simulink model "gm_sampleModel1432_2_sub_sub"  (R2023a)
settings: Solver=VariableStepAuto  StartTime=0.0  StopTime=10.0  RelTol=1e-3
libraries: simulink x1, hdlsllib x1
settings Model: Creator=user1  LastModifiedBy=user1
settings OptimizationCC: BlockReduction=off  ConditionallyExecuteInputs=off
settings DebuggingCC: InheritedTsInSrcMsg=none

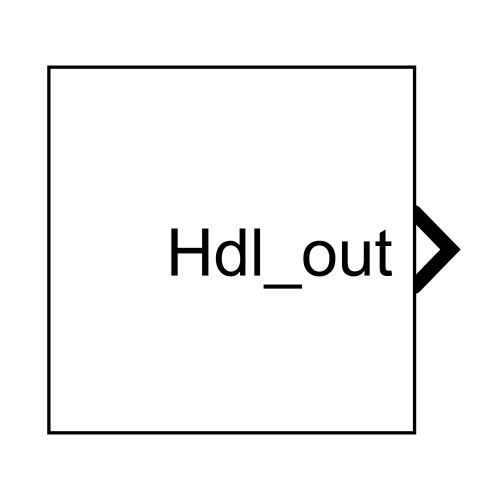
[thumbnail: Simulink's stored preview of the top-level diagram]
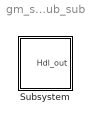
== system gm_sampleModel1432_2_sub_sub ==
  Subsystem : Subsystem

== system gm_sampleModel1432_2_sub_sub/Subsystem ==
  Subsystem : Subsystem
  Hdl_out : Outport  OutDataTypeStr=uint8  SampleTime=1
  wires:
  Subsystem/1(Hdl_out) -> Hdl_out/1

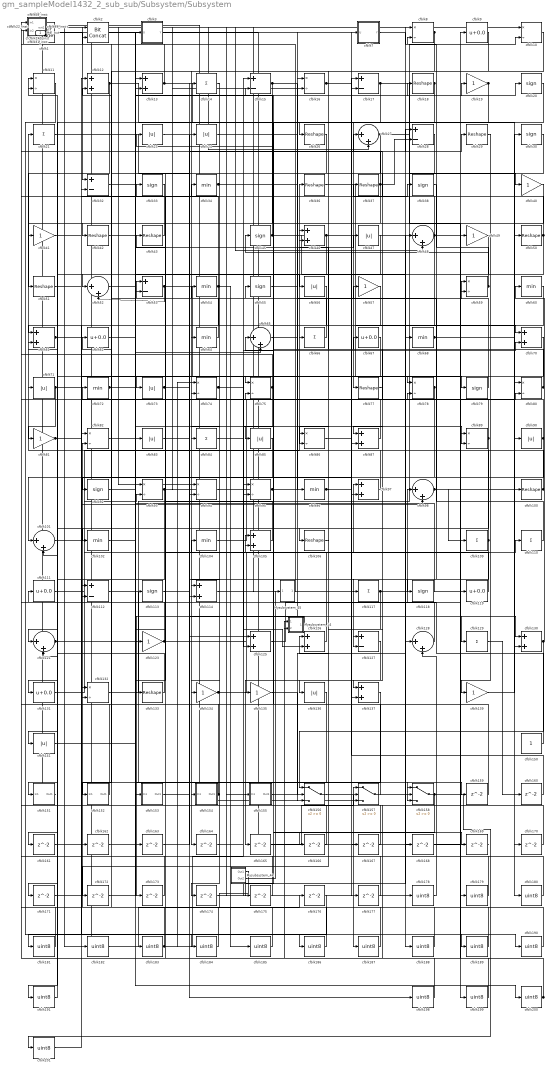
== system gm_sampleModel1432_2_sub_sub/Subsystem/Subsystem ==
  Mysubsystem_14 : Subsystem
  Mysubsystem_44 : Subsystem
  Mysubsystem_45 : Subsystem
  cfblk1 : simulink/Logic and Bit Operations/Detect Change  vinit=0  OutDataTypeStr=uint8
      settings: LibrarySourceBlock=|
      | hdlsllib/Logic and Bit
      | Operations/Detect
      | Change
  cfblk{8,10..11,16,59,74..75,78,80,82,86,89,93..95,132} (16 alike) : Product  Inputs=*/  OutDataTypeStr=uint8  RndMeth=Zero  SaturateOnIntegerOverflow=on
  cfblk{18,26,29,36..37,42..43,50..51,77,100,106,133} (13 alike) : Reshape
  cfblk{27,48,52,65,98,101,121,128} (8 alike) : Sum  Inputs=|++  OutDataTypeStr=uint8
  cfblk{34,54,60,64,68,72,96,102,104} (9 alike) : MinMax  OutDataTypeStr=uint8
  cfblk{12..13,46,61,70,87,97,105,114,125..126,130,137} (13 alike) : Sum  OutDataTypeStr=uint8
  cfblk107_inst : Subsystem
  cfblk108_inst : Subsystem
  cfblk{14,21,66,84,109..110,117,129} (8 alike) : Sum  Inputs=+  OutDataTypeStr=uint8
  cfblk{9,62,67,111,119,131} (6 alike) : Bias  Bias=0.0  SaturateOnIntegerOverflow=off
  cfblk{15,17,28,32,53,112,127} (7 alike) : Sum  Inputs=+-  OutDataTypeStr=uint8
  cfblk{20,30,33,38,45,55,79,92,113,118} (10 alike) : Signum
  cfblk120_inst : Subsystem
  cfblk122_inst : Subsystem
  cfblk{19,40..41,49,57,81,123,134..135,139} (10 alike) : Gain  OutDataTypeStr=uint8
  cfblk{23..24,47,56,71,73,83,85,90,136,141} (11 alike) : Abs  OutDataTypeStr=uint8  SaturateOnIntegerOverflow=off
  cfblk138_inst : Subsystem
  cfblk140_inst : Subsystem
  cfblk150 : Constant  OutDataTypeStr=uint8  SampleTime=-1
  cfblk151 : Subsystem
  cfblk152 : Subsystem
  cfblk153 : Subsystem
  cfblk154 : Subsystem
  cfblk155 : Subsystem
  cfblk156 : Switch  OutDataTypeStr=uint8  SaturateOnIntegerOverflow=off  InputSameDT=off
  cfblk157 : Switch  OutDataTypeStr=uint8  SaturateOnIntegerOverflow=off  InputSameDT=off
  cfblk158 : Switch  OutDataTypeStr=uint8  SaturateOnIntegerOverflow=off  InputSameDT=off
  cfblk{159..177} (19 alike) : Delay  SampleTime=1
  cfblk{178..191,198..201} (18 alike) : DataTypeConversion  OutDataTypeStr=uint8  SaturateOnIntegerOverflow=off  RndMeth=Floor
  cfblk2 : hdlsllib/Logic and Bit Operations/Bit Concat  numInputs=2
  cfblk22_inst : Subsystem
  cfblk3 : Subsystem  mask(Detect Rise Positive){vinit=double(0), InputProcessing=Elements as channels (sample based), OutDataTypeStr=uint8}
      mask prompts: vinit "Simulink:masks:InitialCondition_MP"; InputProcessing "Simulink:masks:InputProcessing_MP"; OutDataTypeStr "Simulink:masks:OutputDataType_MP"
      mask help: Simulink:masks:DetectRisePositive_MD
      mask init:
      | InputProcessing = 'Elements as channels (sample based)';
      | OutDataTypeStr = 'uint8';
      | vinit = double(0);
      mask TypeOptions InputProcessing: Simulink:masks:ColumnsAsChannelsFrameBased | Simulink:masks:ElementsAsChannelsSampleBased
      mask TypeOptions OutDataTypeStr: Simulink:masks:uint8 | Simulink:masks:boolean
      mask Display: fprintf('U > 0\n&  NOT\nU/z > 0')
  cfblk31_inst : Subsystem
  cfblk5 : Constant  Value=0  OutDataTypeStr=uint8  SampleTime=1
  cfblk58_inst : Subsystem
  cfblk7 : Subsystem  mask(Detect Fall Negative){vinit=double(0), InputProcessing=Elements as channels (sample based), OutDataTypeStr=uint8}
      mask prompts: vinit "Simulink:masks:InitialCondition_MP"; InputProcessing "Simulink:masks:InputProcessing_MP"; OutDataTypeStr "Simulink:masks:OutputDataType_MP"
      mask help: Simulink:masks:DetectFallNegative_MD
      mask init:
      | InputProcessing = 'Elements as channels (sample based)';
      | OutDataTypeStr = 'uint8';
      | vinit = double(0);
      mask TypeOptions InputProcessing: Simulink:masks:ColumnsAsChannelsFrameBased | Simulink:masks:ElementsAsChannelsSampleBased
      mask TypeOptions OutDataTypeStr: Simulink:masks:uint8 | Simulink:masks:boolean
      mask Display: fprintf('U < 0\n&  NOT\nU/z < 0')
  cfblk99_inst : Subsystem
  Hdl_out : Outport  OutDataTypeStr=uint8  SampleTime=1
  wires:
  Mysubsystem_14/1(Out1) -> cfblk173/1
  Mysubsystem_44/1(Out1) -> cfblk82/2
  Mysubsystem_44/2(Out2) -> Mysubsystem_45/1(In1)
  Mysubsystem_45/1(Out1) -> cfblk140_inst/2(in2)
  cfblk1/1 -> cfblk32/1
  cfblk10/1 -> cfblk164/1
  cfblk100/1 -> cfblk36/1, cfblk21/1
  cfblk101/1 -> cfblk93/2
  cfblk102/1 -> cfblk3/1(U)
  cfblk104/1 -> cfblk80/2
  cfblk105/1 -> cfblk53/1
  cfblk106/1 -> cfblk126/1
  cfblk107_inst/1(out1) -> cfblk27/2, cfblk119/1
  cfblk108_inst/1(out1) -> cfblk94/1
  cfblk109/1 -> cfblk62/1, cfblk127/2
  cfblk11/1 -> cfblk189/1
  cfblk110/1 -> cfblk55/1
  cfblk111/1 -> cfblk105/1
  cfblk112/1 -> cfblk154/1(In1)
  cfblk113/1 -> cfblk24/1
  cfblk114/1 -> cfblk169/1
  cfblk117/1 -> cfblk136/1, cfblk172/1
  cfblk118/1 -> cfblk93/1
  cfblk119/1 -> cfblk104/1
  cfblk12/1 -> cfblk51/1, cfblk26/1
  cfblk120_inst/1(out1) -> cfblk16/2
  cfblk121/1 -> cfblk15/1, cfblk10/2
  cfblk122_inst/1(out1) -> cfblk96/1
  cfblk123/1 -> cfblk58_inst/1(in1), cfblk110/1
  cfblk125/1 -> cfblk9/1
  cfblk126/1 -> cfblk43/1
  cfblk127/1 -> cfblk165/1
  cfblk128/1 -> cfblk98/1
  cfblk129/1 -> cfblk160/1
  cfblk13/1 -> cfblk90/1, cfblk77/1, cfblk122_inst/2(in2)
  cfblk130/1 -> cfblk156/1, cfblk60/1
  cfblk131/1 -> cfblk66/1
  cfblk132/1 -> cfblk14/1
  cfblk133/1 -> cfblk111/1
  cfblk134/1 -> cfblk97/1, cfblk17/2
  cfblk135/1 -> cfblk158/3
  cfblk136/1 -> cfblk155/1(In1)
  cfblk137/1 -> cfblk163/1
  cfblk138_inst/1(out1) -> cfblk48/2, cfblk49/1
  cfblk139/1 -> cfblk100/1
  cfblk14/1 -> cfblk74/2
  cfblk140_inst/1(out1) -> cfblk182/1, cfblk138_inst/1(in1), cfblk10/1
  cfblk141/1 -> cfblk13/2
  cfblk15/1 -> cfblk130/1, cfblk94/2
  cfblk150/1 -> cfblk112/1
  cfblk151/1(Out1) -> Hdl_out/1
  cfblk152/1(Out1) -> cfblk99_inst/1(in1)
  cfblk153/1(Out1) -> cfblk125/1
  cfblk154/1(Out1) -> cfblk71/1, cfblk72/1
  cfblk155/1(Out1) -> cfblk48/1
  cfblk156/1 -> cfblk187/1
  cfblk157/1 -> cfblk65/1
  cfblk158/1 -> cfblk201/1, cfblk175/1
  cfblk159/1 -> cfblk12/2
  cfblk16/1 -> cfblk89/2, cfblk159/1
  cfblk160/1 -> cfblk17/1
  cfblk161/1 -> cfblk32/2
  cfblk162/1 -> cfblk78/2
  cfblk163/1 -> cfblk80/1
  cfblk164/1 -> cfblk70/2
  cfblk165/1 -> cfblk157/1
  cfblk166/1 -> cfblk53/2
  cfblk167/1 -> cfblk61/2
  cfblk168/1 -> cfblk190/1
  cfblk169/1 -> cfblk1/1
  cfblk17/1 -> cfblk191/1, cfblk40/1
  cfblk170/1 -> cfblk99_inst/2(in2)
  cfblk171/1 -> cfblk98/2
  cfblk172/1 -> cfblk105/2
  cfblk173/1 -> cfblk138_inst/2(in2)
  cfblk174/1 -> cfblk128/1
  cfblk175/1 -> cfblk101/2
  cfblk176/1 -> cfblk181/1
  cfblk177/1 -> cfblk132/1
  cfblk178/1 -> cfblk128/2
  cfblk179/1 -> cfblk22_inst/1(in1)
  cfblk18/1 -> cfblk52/1, cfblk86/2
  cfblk180/1 -> cfblk22_inst/2(in2)
  cfblk181/1 -> cfblk107_inst/2(in2)
  cfblk182/1 -> cfblk176/1
  cfblk183/1 -> cfblk107_inst/1(in1), cfblk95/2, cfblk74/1
  cfblk184/1 -> cfblk31_inst/1(in1)
  cfblk185/1 -> cfblk31_inst/2(in2)
  cfblk186/1 -> cfblk162/1
  cfblk187/1 -> cfblk2/1
  cfblk188/1 -> cfblk2/2
  cfblk189/1 -> cfblk140_inst/1(in1)
  cfblk19/1 -> cfblk75/1, cfblk84/1
  cfblk190/1 -> cfblk11/1
  cfblk191/1 -> cfblk11/2
  cfblk198/1 -> Mysubsystem_14/1(In1)
  cfblk199/1 -> Mysubsystem_14/2(In2)
  cfblk2/1 -> cfblk186/1
  cfblk20/1 -> cfblk174/1
  cfblk200/1 -> cfblk33/1, cfblk157/2, cfblk122_inst/1(in1), cfblk89/1
  cfblk201/1 -> cfblk82/1
  cfblk21/1 -> cfblk114/2
  cfblk22_inst/1(out1) -> cfblk178/1
  cfblk23/1 -> cfblk78/1
  cfblk24/1 -> cfblk20/1
  cfblk26/1 -> cfblk134/1
  cfblk27/1 -> cfblk42/1, cfblk199/1
  cfblk28/1 -> cfblk87/1
  cfblk29/1 -> cfblk139/1
  cfblk3/1(Y) -> cfblk177/1
  cfblk30/1 -> cfblk73/1
  cfblk31_inst/1(out1) -> cfblk183/1
  cfblk32/1 -> cfblk56/1
  cfblk33/1 -> cfblk92/1
  cfblk34/1 -> cfblk114/1, cfblk170/1
  cfblk36/1 -> cfblk70/1
  cfblk37/1 -> cfblk61/1, cfblk28/2, cfblk108_inst/1(in1)
  cfblk38/1 -> cfblk118/1
  cfblk40/1 -> cfblk123/1
  cfblk41/1 -> cfblk12/1
  cfblk42/1 -> cfblk158/1
  cfblk43/1 -> cfblk41/1
  cfblk45/1 -> cfblk13/1, cfblk168/1
  cfblk46/1 -> cfblk188/1, cfblk152/1(In1)
  cfblk47/1 -> cfblk141/1
  cfblk48/1 -> cfblk37/1, cfblk8/2, cfblk171/1
  cfblk49/1 -> cfblk85/1
  cfblk5/1 -> cfblk157/3
  cfblk50/1 -> cfblk27/1, cfblk135/1
  cfblk51/1 -> cfblk38/1
  cfblk52/1 -> cfblk86/1
  cfblk53/1 -> cfblk52/2, cfblk95/1
  cfblk54/1 -> cfblk185/1, cfblk120_inst/2(in2), cfblk112/2
  cfblk55/1 -> cfblk87/2
  cfblk56/1 -> cfblk64/1
  cfblk57/1 -> cfblk106/1
  cfblk58_inst/1(out1) -> cfblk83/1
  cfblk59/1 -> cfblk45/1, cfblk8/1
  cfblk60/1 -> cfblk137/1
  cfblk61/1 -> cfblk79/1, cfblk34/1
  cfblk62/1 -> cfblk113/1
  cfblk64/1 -> cfblk54/1
  cfblk65/1 -> cfblk179/1
  cfblk66/1 -> cfblk108_inst/2(in2)
  cfblk67/1 -> cfblk161/1
  cfblk68/1 -> cfblk50/1, cfblk180/1
  cfblk7/1(Y) -> cfblk68/1
  cfblk70/1 -> cfblk133/1
  cfblk71/1 -> cfblk81/1, cfblk75/2, cfblk153/1(In1)
  cfblk72/1 -> cfblk65/2, cfblk47/1
  cfblk73/1 -> cfblk198/1, cfblk117/1
  cfblk74/1 -> cfblk29/1, cfblk19/1
  cfblk75/1 -> cfblk58_inst/2(in2), cfblk125/2
  cfblk77/1 -> cfblk127/1
  cfblk78/1 -> cfblk156/3, cfblk121/2, cfblk132/2
  cfblk79/1 -> cfblk59/1
  cfblk8/1 -> cfblk156/2, cfblk137/2
  cfblk80/1 -> cfblk46/1, cfblk23/1
  cfblk81/1 -> cfblk97/2, cfblk184/1
  cfblk82/1 -> cfblk200/1
  cfblk83/1 -> cfblk28/1
  cfblk84/1 -> cfblk126/2
  cfblk85/1 -> cfblk101/1
  cfblk86/1 -> cfblk59/2
  cfblk87/1 -> cfblk120_inst/1(in1)
  cfblk89/1 -> cfblk67/1, cfblk131/1
  cfblk9/1 -> cfblk102/1
  cfblk90/1 -> cfblk121/1, cfblk16/1
  cfblk92/1 -> cfblk18/1
  cfblk93/1 -> cfblk46/2, cfblk130/2, cfblk151/1(In1)
  cfblk94/1 -> cfblk129/1
  cfblk95/1 -> cfblk57/1, cfblk7/1(U)
  cfblk96/1 -> cfblk167/1, cfblk166/1
  cfblk97/1 -> cfblk15/2
  cfblk98/1 -> cfblk30/1, cfblk109/1
  cfblk99_inst/1(out1) -> cfblk158/2

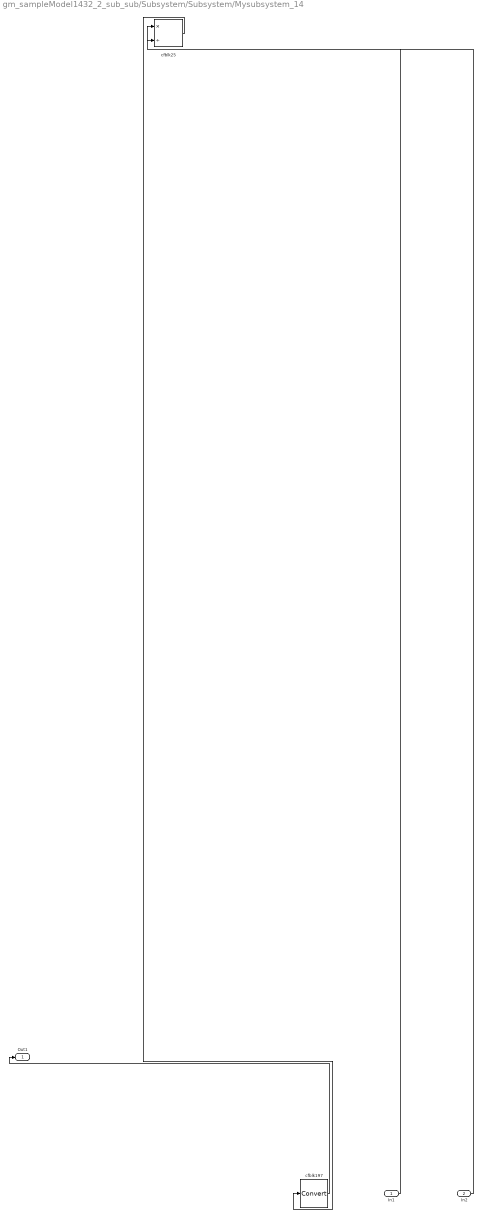
== system gm_sampleModel1432_2_sub_sub/Subsystem/Subsystem/Mysubsystem_14 ==
  In1 : Inport  OutDataTypeStr=uint8  PortDimensions=1  SampleTime=1
  In2 : Inport  Port=2  OutDataTypeStr=uint8  PortDimensions=1  SampleTime=1
  cfblk197 : DataTypeConversion  SaturateOnIntegerOverflow=off  RndMeth=Floor
  cfblk25 : Product  Inputs=*/  RndMeth=Zero  SaturateOnIntegerOverflow=on
  Out1 : Outport  SampleTime=1
  wires:
  In1/1 -> cfblk25/1
  In2/1 -> cfblk25/2
  cfblk197/1 -> Out1/1
  cfblk25/1 -> cfblk197/1

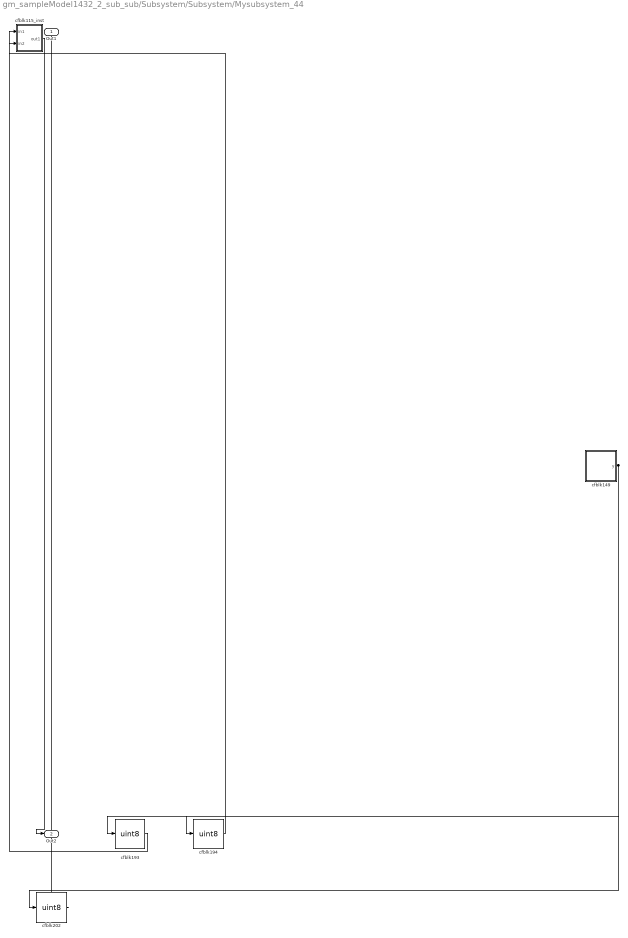
== system gm_sampleModel1432_2_sub_sub/Subsystem/Subsystem/Mysubsystem_44 ==
  cfblk115_inst : Subsystem
  cfblk149 : Subsystem  mask(Counter Limited){uplimit=double(7), tsamp=double(-1)}
      mask prompts: uplimit "Simulink:masks:UpperLimit_MP"; tsamp "Simulink:masks:SampleTime_MP"
      mask help: Simulink:masks:CounterLimited_MD
      mask init:
      | nbits = double(8);
      | tsamp = double(-1);
      | uplimit = double(7);
  cfblk193 : DataTypeConversion  OutDataTypeStr=uint8  SaturateOnIntegerOverflow=off  RndMeth=Floor
  cfblk194 : DataTypeConversion  OutDataTypeStr=uint8  SaturateOnIntegerOverflow=off  RndMeth=Floor
  cfblk202 : DataTypeConversion  OutDataTypeStr=uint8  SaturateOnIntegerOverflow=off  RndMeth=Floor
  Out1 : Outport  SampleTime=1
  Out2 : Outport  Port=2  SampleTime=1
  wires:
  cfblk115_inst/1(out1) -> Out2/1
  cfblk149/1(y) -> cfblk202/1, cfblk194/1, cfblk193/1
  cfblk193/1 -> cfblk115_inst/1(in1)
  cfblk194/1 -> cfblk115_inst/2(in2)
  cfblk202/1 -> Out1/1

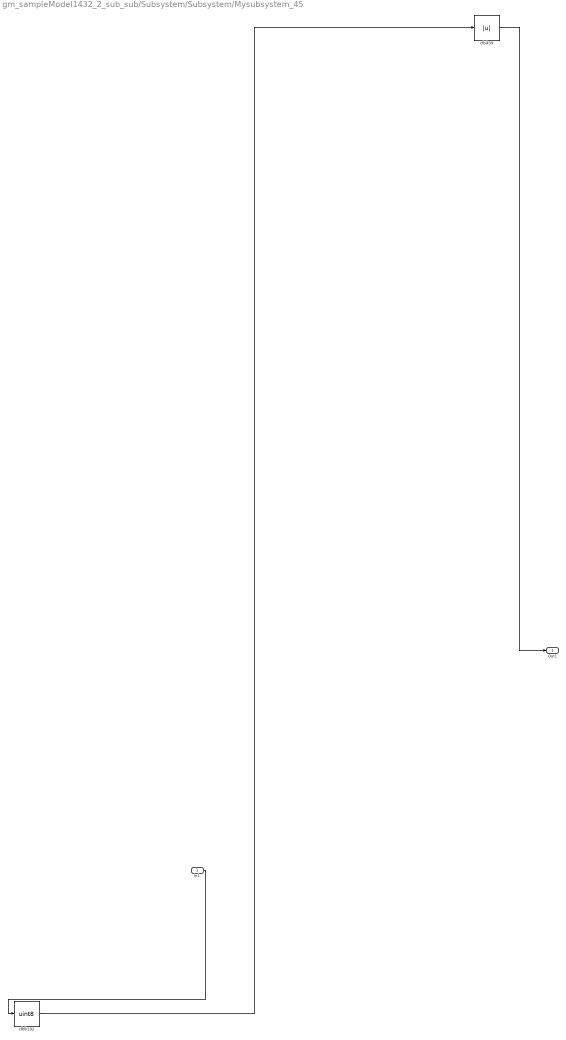
== system gm_sampleModel1432_2_sub_sub/Subsystem/Subsystem/Mysubsystem_45 ==
  In1 : Inport  OutDataTypeStr=uint16  PortDimensions=1  SampleTime=1
  cfblk192 : DataTypeConversion  OutDataTypeStr=uint8  SaturateOnIntegerOverflow=off  RndMeth=Floor
  cfblk39 : Abs  SaturateOnIntegerOverflow=off
  Out1 : Outport  SampleTime=1
  wires:
  In1/1 -> cfblk192/1
  cfblk192/1 -> cfblk39/1
  cfblk39/1 -> Out1/1

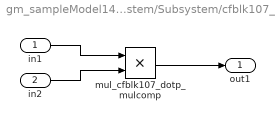
== system gm_sampleModel1432_2_sub_sub/Subsystem/Subsystem/cfblk107_inst ==
  in1 : Inport  OutDataTypeStr=uint8  SampleTime=1
  in2 : Inport  Port=2  OutDataTypeStr=uint8  SampleTime=1
  mul_cfblk107_dotp_mulcomp : Product  Inputs=**  OutDataTypeStr=uint8  SampleTime=1
  out1 : Outport  OutDataTypeStr=uint8  SampleTime=1
  wires:
  in1/1 -> mul_cfblk107_dotp_mulcomp/1
  in2/1 -> mul_cfblk107_dotp_mulcomp/2
  mul_cfblk107_dotp_mulcomp/1 -> out1/1

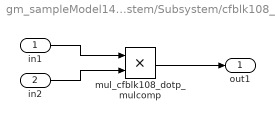
== system gm_sampleModel1432_2_sub_sub/Subsystem/Subsystem/cfblk108_inst ==
  in1 : Inport  OutDataTypeStr=uint8  SampleTime=1
  in2 : Inport  Port=2  OutDataTypeStr=uint8  SampleTime=1
  mul_cfblk108_dotp_mulcomp : Product  Inputs=**  OutDataTypeStr=uint8  SampleTime=1
  out1 : Outport  OutDataTypeStr=uint8  SampleTime=1
  wires:
  in1/1 -> mul_cfblk108_dotp_mulcomp/1
  in2/1 -> mul_cfblk108_dotp_mulcomp/2
  mul_cfblk108_dotp_mulcomp/1 -> out1/1

== system gm_sampleModel1432_2_sub_sub/Subsystem/Subsystem/cfblk120_inst ==
  in1 : Inport  OutDataTypeStr=uint8  SampleTime=1
  in2 : Inport  Port=2  OutDataTypeStr=uint8  SampleTime=1
  mul_cfblk120_dotp_mulcomp : Product  Inputs=**  OutDataTypeStr=uint8  SampleTime=1
  out1 : Outport  OutDataTypeStr=uint8  SampleTime=1
  wires:
  in1/1 -> mul_cfblk120_dotp_mulcomp/1
  in2/1 -> mul_cfblk120_dotp_mulcomp/2
  mul_cfblk120_dotp_mulcomp/1 -> out1/1

== system gm_sampleModel1432_2_sub_sub/Subsystem/Subsystem/cfblk122_inst ==
  in1 : Inport  OutDataTypeStr=uint8  SampleTime=1
  in2 : Inport  Port=2  OutDataTypeStr=uint8  SampleTime=1
  mul_cfblk122_dotp_mulcomp : Product  Inputs=**  OutDataTypeStr=uint8  SampleTime=1
  out1 : Outport  OutDataTypeStr=uint8  SampleTime=1
  wires:
  in1/1 -> mul_cfblk122_dotp_mulcomp/1
  in2/1 -> mul_cfblk122_dotp_mulcomp/2
  mul_cfblk122_dotp_mulcomp/1 -> out1/1

== system gm_sampleModel1432_2_sub_sub/Subsystem/Subsystem/cfblk138_inst ==
  in1 : Inport  OutDataTypeStr=uint8  SampleTime=1
  in2 : Inport  Port=2  OutDataTypeStr=uint8  SampleTime=1
  mul_cfblk138_dotp_mulcomp : Product  Inputs=**  OutDataTypeStr=uint8  SampleTime=1
  out1 : Outport  OutDataTypeStr=uint8  SampleTime=1
  wires:
  in1/1 -> mul_cfblk138_dotp_mulcomp/1
  in2/1 -> mul_cfblk138_dotp_mulcomp/2
  mul_cfblk138_dotp_mulcomp/1 -> out1/1

== system gm_sampleModel1432_2_sub_sub/Subsystem/Subsystem/cfblk140_inst ==
  in1 : Inport  OutDataTypeStr=uint8  SampleTime=1
  in2 : Inport  Port=2  OutDataTypeStr=uint8  SampleTime=1
  mul_cfblk140_dotp_mulcomp : Product  Inputs=**  OutDataTypeStr=uint8  SampleTime=1
  out1 : Outport  OutDataTypeStr=uint8  SampleTime=1
  wires:
  in1/1 -> mul_cfblk140_dotp_mulcomp/1
  in2/1 -> mul_cfblk140_dotp_mulcomp/2
  mul_cfblk140_dotp_mulcomp/1 -> out1/1

== system gm_sampleModel1432_2_sub_sub/Subsystem/Subsystem/cfblk151 ==
  In1 : Inport  OutDataTypeStr=uint8  PortDimensions=1  SampleTime=1
  Out1 : Outport  SampleTime=1
  wires:
  In1/1 -> Out1/1

== system gm_sampleModel1432_2_sub_sub/Subsystem/Subsystem/cfblk152 ==
  In1 : Inport  OutDataTypeStr=uint8  PortDimensions=1  SampleTime=1
  Out1 : Outport  SampleTime=1
  wires:
  In1/1 -> Out1/1

== system gm_sampleModel1432_2_sub_sub/Subsystem/Subsystem/cfblk153 ==
  In1 : Inport  OutDataTypeStr=uint8  PortDimensions=1  SampleTime=1
  Out1 : Outport  SampleTime=1
  wires:
  In1/1 -> Out1/1

== system gm_sampleModel1432_2_sub_sub/Subsystem/Subsystem/cfblk154 ==
  In1 : Inport  OutDataTypeStr=uint8  PortDimensions=1  SampleTime=1
  Out1 : Outport  SampleTime=1
  wires:
  In1/1 -> Out1/1

== system gm_sampleModel1432_2_sub_sub/Subsystem/Subsystem/cfblk155 ==
  In1 : Inport  OutDataTypeStr=uint8  PortDimensions=1  SampleTime=1
  Out1 : Outport  SampleTime=1
  wires:
  In1/1 -> Out1/1

== system gm_sampleModel1432_2_sub_sub/Subsystem/Subsystem/cfblk22_inst ==
  in1 : Inport  OutDataTypeStr=uint8  SampleTime=1
  in2 : Inport  Port=2  OutDataTypeStr=uint8  SampleTime=1
  mul_cfblk22_dotp_mulcomp : Product  Inputs=**  OutDataTypeStr=uint8  SampleTime=1
  out1 : Outport  OutDataTypeStr=uint8  SampleTime=1
  wires:
  in1/1 -> mul_cfblk22_dotp_mulcomp/1
  in2/1 -> mul_cfblk22_dotp_mulcomp/2
  mul_cfblk22_dotp_mulcomp/1 -> out1/1

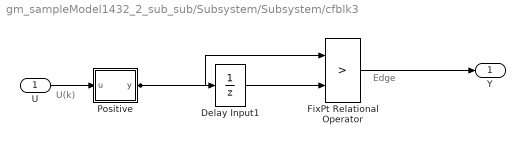
== system gm_sampleModel1432_2_sub_sub/Subsystem/Subsystem/cfblk3 ==
  note: U(k)
  note: Edge
  U : Inport  OutDataTypeStr=uint8  SampleTime=1
  Delay Input1 : UnitDelay  Description=Store in Global RAM  DisableCoverage=on  InitialCondition=vinit  SampleTime=-1  HasFrameUpgradeWarning=on
  FixPt Relational Operator : RelationalOperator  Operator=>  OutDataTypeStr=fixdt(0, 8)  ZeroCross=off  InputSameDT=off
  Positive : Subsystem  mask(Compare To Zero){relop=>, OutDataTypeStr=boolean, ZeroCross=off}
      mask prompts: relop "Simulink:masks:Operator_MP"; OutDataTypeStr "Simulink:masks:OutputDataType_MP"; ZeroCross "Simulink:masks:EnableZerocrossingDetection_MP"
      mask help: Simulink:masks:CompareToZero_MD
      mask init:
      | OutDataTypeStr = 'boolean';
      | ZeroCross = 'off';
      | blkName = 'sampleModel1432_2_sub_sub/Subsystem/Subsystem/cfblk3/Positive';
      | relop = '>';
      | setValue = 'boolean';
      mask TypeOptions relop: == | ~= | < | <= | >= | >
      mask TypeOptions OutDataTypeStr: Simulink:masks:uint8 | Simulink:masks:boolean
      mask Callback ZeroCross: sl('zeroCrossEnable', gcbh);
      mask Display: disp([relop,' 0'])
  Y : Outport  SampleTime=1
  wires:
  U/1 -> Positive/1(u)
  Delay Input1/1 -> FixPt Relational Operator/2
  FixPt Relational Operator/1 -> Y/1
  Positive/1(y) -> FixPt Relational Operator/1, Delay Input1/1

== system gm_sampleModel1432_2_sub_sub/Subsystem/Subsystem/cfblk31_inst ==
  in1 : Inport  OutDataTypeStr=uint8  SampleTime=1
  in2 : Inport  Port=2  OutDataTypeStr=uint8  SampleTime=1
  mul_cfblk31_dotp_mulcomp : Product  Inputs=**  OutDataTypeStr=uint8  SampleTime=1
  out1 : Outport  OutDataTypeStr=uint8  SampleTime=1
  wires:
  in1/1 -> mul_cfblk31_dotp_mulcomp/1
  in2/1 -> mul_cfblk31_dotp_mulcomp/2
  mul_cfblk31_dotp_mulcomp/1 -> out1/1

== system gm_sampleModel1432_2_sub_sub/Subsystem/Subsystem/cfblk58_inst ==
  in1 : Inport  OutDataTypeStr=uint8  SampleTime=1
  in2 : Inport  Port=2  OutDataTypeStr=uint8  SampleTime=1
  mul_cfblk58_dotp_mulcomp : Product  Inputs=**  OutDataTypeStr=uint8  SampleTime=1
  out1 : Outport  OutDataTypeStr=uint8  SampleTime=1
  wires:
  in1/1 -> mul_cfblk58_dotp_mulcomp/1
  in2/1 -> mul_cfblk58_dotp_mulcomp/2
  mul_cfblk58_dotp_mulcomp/1 -> out1/1

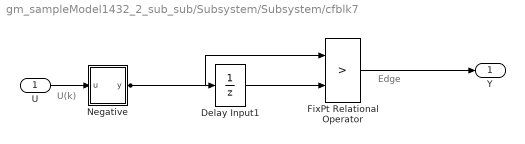
== system gm_sampleModel1432_2_sub_sub/Subsystem/Subsystem/cfblk7 ==
  note: U(k)
  note: Edge
  U : Inport  OutDataTypeStr=uint8  SampleTime=1
  Delay Input1 : UnitDelay  Description=Store in Global RAM  DisableCoverage=on  InitialCondition=vinit  SampleTime=-1  HasFrameUpgradeWarning=on
  FixPt Relational Operator : RelationalOperator  Operator=>  OutDataTypeStr=fixdt(0, 8)  ZeroCross=off  InputSameDT=off
  Negative : Subsystem  mask(Compare To Zero){relop=<, OutDataTypeStr=boolean, ZeroCross=off}
      mask prompts: relop "Simulink:masks:Operator_MP"; OutDataTypeStr "Simulink:masks:OutputDataType_MP"; ZeroCross "Simulink:masks:EnableZerocrossingDetection_MP"
      mask help: Simulink:masks:CompareToZero_MD
      mask init:
      | OutDataTypeStr = 'boolean';
      | ZeroCross = 'off';
      | blkName = 'sampleModel1432_2_sub_sub/Subsystem/Subsystem/cfblk7/Negative';
      | relop = '<';
      | setValue = 'boolean';
      mask TypeOptions relop: == | ~= | < | <= | >= | >
      mask TypeOptions OutDataTypeStr: Simulink:masks:uint8 | Simulink:masks:boolean
      mask Callback ZeroCross: sl('zeroCrossEnable', gcbh);
      mask Display: disp([relop,' 0'])
  Y : Outport  SampleTime=1
  wires:
  U/1 -> Negative/1(u)
  Delay Input1/1 -> FixPt Relational Operator/2
  FixPt Relational Operator/1 -> Y/1
  Negative/1(y) -> FixPt Relational Operator/1, Delay Input1/1

== system gm_sampleModel1432_2_sub_sub/Subsystem/Subsystem/cfblk99_inst ==
  in1 : Inport  OutDataTypeStr=uint8  SampleTime=1
  in2 : Inport  Port=2  OutDataTypeStr=uint8  SampleTime=1
  mul_cfblk99_dotp_mulcomp : Product  Inputs=**  OutDataTypeStr=uint8  SampleTime=1
  out1 : Outport  OutDataTypeStr=uint8  SampleTime=1
  wires:
  in1/1 -> mul_cfblk99_dotp_mulcomp/1
  in2/1 -> mul_cfblk99_dotp_mulcomp/2
  mul_cfblk99_dotp_mulcomp/1 -> out1/1

== system gm_sampleModel1432_2_sub_sub/Subsystem/Subsystem/Mysubsystem_44/cfblk115_inst ==
  in1 : Inport  OutDataTypeStr=uint8  SampleTime=1
  in2 : Inport  Port=2  OutDataTypeStr=uint8  SampleTime=1
  mul_cfblk115_dotp_mulcomp : Product  Inputs=**  OutDataTypeStr=uint16  SampleTime=1
  out1 : Outport  OutDataTypeStr=uint16  SampleTime=1
  wires:
  in1/1 -> mul_cfblk115_dotp_mulcomp/1
  in2/1 -> mul_cfblk115_dotp_mulcomp/2
  mul_cfblk115_dotp_mulcomp/1 -> out1/1

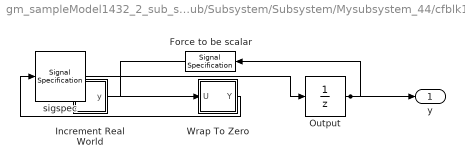
== system gm_sampleModel1432_2_sub_sub/Subsystem/Subsystem/Mysubsystem_44/cfblk149 ==
  Force to be scalar : SignalSpecification  DisableCoverage=on  Dimensions=1
  Increment Real World : Subsystem  mask(Real World Value Increment){}
      mask help: Simulink:masks:RealWorldValueIncrement_MD
      mask Display: disp('V++')
  Output : UnitDelay  InitialCondition=0.0  SampleTime=tsamp  HasFrameUpgradeWarning=on
  Wrap To Zero : Subsystem  mask(Wrap To Zero){Threshold=double(7)}
      mask prompts: Threshold "Simulink:masks:Threshold_MP"
      mask help: Simulink:masks:WrapToZero_MD
  sigspec : SignalSpecification  OutDataTypeStr=uint8  Dimensions=1
  y : Outport  SampleTime=1
  wires:
  Force to be scalar/1 -> Increment Real World/1(u)
  Increment Real World/1(y) -> Wrap To Zero/1(U)
  Output/1 -> Force to be scalar/1, y/1
  Wrap To Zero/1(Y) -> sigspec/1
  sigspec/1 -> Output/1

== system gm_sampleModel1432_2_sub_sub/Subsystem/Subsystem/cfblk3/Positive ==
  u : Inport  OutDataTypeStr=uint8  SampleTime=1
  Compare : RelationalOperator  Operator=>  OutDataTypeStr=boolean  ZeroCross=off
  Constant : Constant  DisableCoverage=on  Value=0  OutDataTypeStr=Inherit: Inherit via back propagation  SampleTime=-1  PreserveConstantTs=on
  y : Outport  SampleTime=1
  wires:
  u/1 -> Compare/1
  Compare/1 -> y/1
  Constant/1 -> Compare/2

== system gm_sampleModel1432_2_sub_sub/Subsystem/Subsystem/cfblk7/Negative ==
  u : Inport  OutDataTypeStr=uint8  SampleTime=1
  Compare : RelationalOperator  Operator=<  OutDataTypeStr=boolean  ZeroCross=off
  Constant : Constant  DisableCoverage=on  Value=0  OutDataTypeStr=Inherit: Inherit via back propagation  SampleTime=-1  PreserveConstantTs=on
  y : Outport  SampleTime=1
  wires:
  u/1 -> Compare/1
  Compare/1 -> y/1
  Constant/1 -> Compare/2

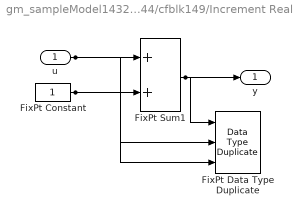
== system gm_sampleModel1432_2_sub_sub/Subsystem/Subsystem/Mysubsystem_44/cfblk149/Increment Real World ==
  u : Inport  OutDataTypeStr=uint8  SampleTime=1
  FixPt Constant : Constant  DisableCoverage=on  OutDataTypeStr=Inherit: Inherit via back propagation  SampleTime=-1
  FixPt Data Type Duplicate : DataTypeDuplicate  DisableCoverage=on  NumInputPorts=3
  FixPt Sum1 : Sum  InputSameDT=on  OutDataTypeStr=Inherit: Inherit via back propagation  LockScale=on
  y : Outport  SampleTime=1
  wires:
  u/1 -> FixPt Sum1/1, FixPt Data Type Duplicate/2
  FixPt Constant/1 -> FixPt Sum1/2, FixPt Data Type Duplicate/3
  FixPt Sum1/1 -> FixPt Data Type Duplicate/1, y/1

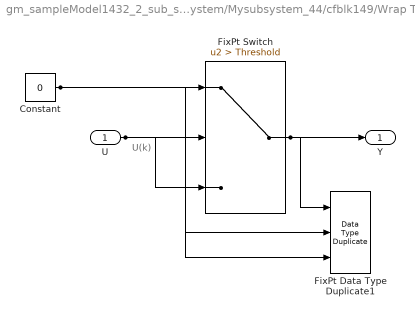
== system gm_sampleModel1432_2_sub_sub/Subsystem/Subsystem/Mysubsystem_44/cfblk149/Wrap To Zero ==
  note: U(k)
  U : Inport  OutDataTypeStr=uint8  SampleTime=1
  Constant : Constant  DisableCoverage=on  Value=0  OutDataTypeStr=Inherit: Inherit via back propagation  SampleTime=-1
  FixPt Data Type Duplicate1 : DataTypeDuplicate  DisableCoverage=on  NumInputPorts=3
  FixPt Switch : Switch  Criteria=u2 > Threshold  Threshold=Threshold  OutDataTypeStr=Inherit: Inherit via back propagation  ZeroCross=off  SaturateOnIntegerOverflow=off  InputSameDT=off
  Y : Outport  SampleTime=1
  wires:
  U/1 -> FixPt Switch/3, FixPt Switch/2, FixPt Data Type Duplicate1/2
  Constant/1 -> FixPt Switch/1, FixPt Data Type Duplicate1/3
  FixPt Switch/1 -> FixPt Data Type Duplicate1/1, Y/1
